simulink model "Figure_2_3_TP_Telecom_modulation_demodulation_ASK2_bis"  (R2020a)
settings: Solver=VariableStepAuto  StartTime=0.0  StopTime=10.0  RelTol=1e-3
undefined symbols (not defined in the file or in its folder): fdesignblkfcn, gcbh
libraries: simulink x2, dspsrcs4 x2, commrandsrc3 x1, dsparch4 x1, commsink2 x1, commfilt2 x1, dspsigops x1, commutil2 x1
settings Model: Creator=iba  LastModifiedBy=iba

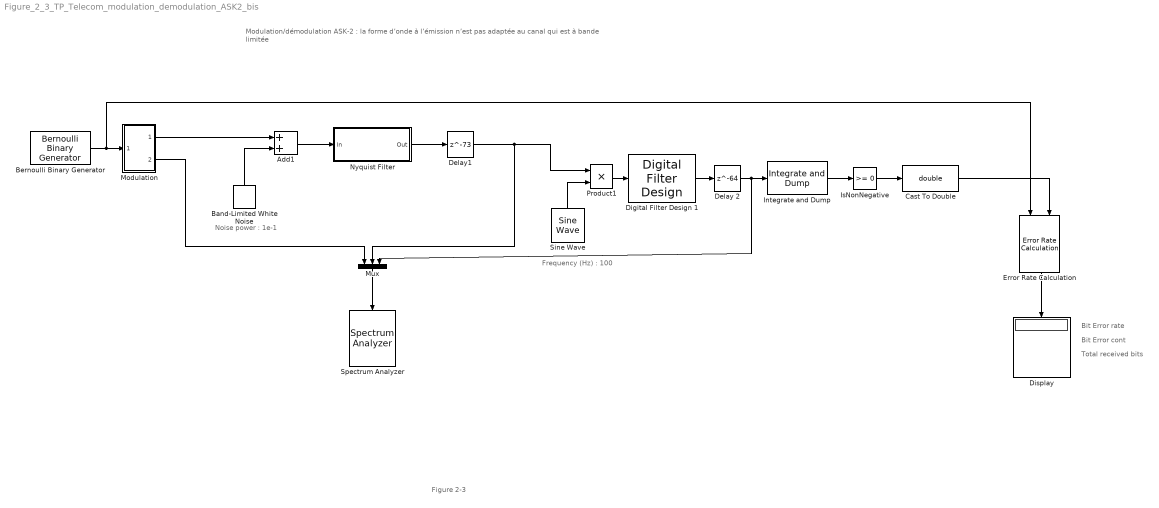
== system Figure_2_3_TP_Telecom_modulation_demodulation_ASK2_bis ==
  note: Figure 2-3
  note: Noise power : 1e-1
  note: Modulation/démodulation ASK-2 : la forme d’onde à l’émission n’est pas adaptée au canal qui est à bande limitée
  note: Frequency (Hz) : 100
  note: Bit Error rate
  note: Bit Error cont
  note: Total received bits
  Add1 : Sum
  "Band-Limited White Noise " : simulink/Sources/Band-Limited White Noise  Cov=[1e-1]  Ts=1  seed=[1]
  "Bernoulli Binary Generator " : commrandsrc3/Bernoulli Binary Generator  ProbabilityOfZero=0.5  SeedSource=Parameter  Seed=25.  SampleTime=0.01  SamplesPerFrame=1  OutputDataType=double  SimulateUsing=Interpreted execution
  Cast To Double : DataTypeConversion  OutDataTypeStr=double
  Delay 2 : Delay  DelayLength=64  InitialCondition=0
  "Delay1 " : Delay  DelayLength=73  InitialCondition=0
  Digital Filter Design 1 : dsparch4/Digital Filter Design  mwdsp_browser_bugfix_var=off
  "Display " : Display
  Error Rate Calculation : commsink2/Error Rate Calculation  N=1  st_delay=0  cp_mode=Entire frame  subframe=[]  PMode=Port  WsName=ErrorVec  RsMode2=off  stop=off  numErr=100  maxBits=1e6
  Integrate and Dump : commfilt2/Integrate and Dump  obssamples=2  offsetsamples=0  nodump=off  roundingMode=Floor  overflowMode=off
  IsNonNegative : simulink/Logic and Bit Operations/Compare To Zero  relop=>=  OutDataTypeStr=boolean
  Modulation : Subsystem
  Mux : Mux  Inputs=3
  Nyquist Filter : Subsystem  DialogController=fdesignblkfcn  InitFcn=fdesignblkfcn(gcbh, {'InitFcn'});  mask(Nyquist Filter){}
      mask help: Design a Nyquist filter
      settings: CopyFcn=fdesignblkfcn(gcbh, {'CopyFcn'});
      mask Help: helpview(mapfilelocation('dsp'), 'dspnyquistfilter');
      mask Display: disp('Nyquist');
  "Product1 " : Product
  Sine Wave : dspsrcs4/Sine Wave  Amplitude=1  Frequency=100  Phase=0  SampleMode=Discrete  OutComplex=Real  CompMethod=Trigonometric fcn  TableSize=Speed  SampleTime=1  SamplesPerFrame=1  ResetState=Restart at time zero  OutputFrames=off  dataType=double  wordLen=16  udDataType=sfix(16)  fracBitsMode=Best precision  numFracBits=15  OutDataTypeStr=double  LastOutDataTypeStr=double
  "Spectrum Analyzer " : SpectrumAnalyzer
  wires:
  "Bernoulli Binary Generator "/1 -> Modulation/1(IN1), Error Rate Calculation/1
  "Band-Limited White Noise "/1 -> Add1/2
  Sine Wave/1 -> "Product1 "/2
  Add1/1 -> Nyquist Filter/1(In)
  Nyquist Filter/1(Out) -> "Delay1 "/1
  Mux/1 -> "Spectrum Analyzer "/1
  "Delay1 "/1 -> Mux/2, "Product1 "/1
  Cast To Double/1 -> Error Rate Calculation/2
  Integrate and Dump/1 -> IsNonNegative/1
  IsNonNegative/1 -> Cast To Double/1
  Error Rate Calculation/1 -> "Display "/1
  Modulation/1(OUT1) -> Add1/1
  Modulation/2(OUT2) -> Mux/1
  "Product1 "/1 -> Digital Filter Design 1/1
  Digital Filter Design 1/1 -> Delay 2/1
  Delay 2/1 -> Mux/3, Integrate and Dump/1

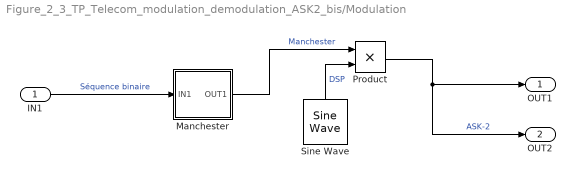
== system Figure_2_3_TP_Telecom_modulation_demodulation_ASK2_bis/Modulation ==
  IN1 : Inport
  Manchester : Subsystem
  "Product " : Product  OutDataTypeStr=double  LockScale=on
  Sine Wave : dspsrcs4/Sine Wave  Amplitude=1  Frequency=5  Phase=0  SampleMode=Discrete  OutComplex=Real  CompMethod=Trigonometric fcn  TableSize=Speed  SampleTime=1  SamplesPerFrame=1  ResetState=Restart at time zero  OutputFrames=off  dataType=Inherit via back propagation  wordLen=16  udDataType=sfix(16)  fracBitsMode=Best precision  numFracBits=15  OutDataTypeStr=Inherit: Inherit via back propagation  LastOutDataTypeStr=Inherit: Inherit via back propagation
  OUT1 : Outport
  OUT2 : Outport  Port=2
  wires:
  "Product "/1 -> OUT2/1, OUT1/1  "ASK-2"
  Sine Wave/1 -> "Product "/2  "DSP"
  Manchester/1(OUT1) -> "Product "/1  "Manchester"
  IN1/1 -> Manchester/1(IN1)  "Séquence binaire"

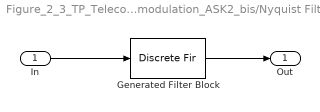
== system Figure_2_3_TP_Telecom_modulation_demodulation_ASK2_bis/Nyquist Filter ==
  In : Inport
  Generated Filter Block : DiscreteFir  Tag=BlockMethodSubSystem  Coefficients=[-1.51622726129955863e-05 0 4.17065642797130267e-05 0 -8.63974532359493069e-05 0 0.000156112339412392586 0 -0.000259152163405612895 0 0.000405340967727107018 0 -0.000606122081126900724 0 0.000874664613518894908 0 -0.00122600321576426152 0 0.00167724728876562468 0 -0.00224791534173759749 0 0.00296048017608780203 0 -0.00384125870473808143 0 0.00492186111131599595 0 -0.00624155643186620392 0 0.00785117446710228636 0 -0.00981967458384361454 0 0.0122455627766693432 0 -0.0152776505052993374 0 0.0191551639220552683 0 -0.0242917549435244136 0 0.0314715991488982369 0 -0.0423816072426853388 0 0.0614206608292716463 0 -0.104744991792953324 0 0.317854846111936151 0.5 0.317854846111936151 0 -0.104744991792953324 0 0.0614206608292716463 0 -0.0423816072426853388 0 0.0314715991488982369 0 -0.0242917549435244136 0 0.0191551639220552683 0 -0.0152776505052993374 0 0.0122455627766693432 0 -0.00981967458384361454 0 0.00785117446710228636 0 -0.00624155643186620392 0 0.00492186111131599595 0 -0.00384125870473808143 0 0.00296048017608780203 0 -0.00224791534173759749 0 0.00167724728876562468 0 -0.00122600321576426152 0 0.000874664613518894908 0 -0.000606122081126900724 0 0.000405340967727107018 0 -0.000259152163405612895 0 0.000156112339412392586 0 -8.63974532359493069e-05 0 4.17065642797130267e-05 0 -1.51622726129955863e-05]  InputProcessing=Columns as channels (frame based)
  Out : Outport  VectorParamsAs1DForOutWhenUnconnected=off
  wires:
  In/1 -> Generated Filter Block/1
  Generated Filter Block/1 -> Out/1

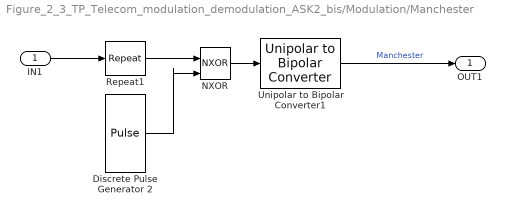
== system Figure_2_3_TP_Telecom_modulation_demodulation_ASK2_bis/Modulation/Manchester ==
  IN1 : Inport
  "Discrete Pulse Generator 2  " : DiscretePulseGenerator  SampleTime=0.01
  "NXOR " : Logic  Operator=NXOR  IconShape=distinctive  AllPortsSameDT=off  OutDataTypeStr=boolean
  Repeat1 : dspsigops/Repeat  N=2  InputProcessing=Columns as channels (frame based)  RateOptions=Enforce single-rate processing  ic=0  mode=Unused parameter value
  Unipolar to Bipolar Converter1 : commutil2/Unipolar to Bipolar Converter  M=2  polarity=Positive  dataType=double
  OUT1 : Outport
  wires:
  IN1/1 -> Repeat1/1
  "NXOR "/1 -> Unipolar to Bipolar Converter1/1
  "Discrete Pulse Generator 2  "/1 -> "NXOR "/2
  Unipolar to Bipolar Converter1/1 -> OUT1/1  "Manchester"
  Repeat1/1 -> "NXOR "/1
